simulink model "hw1_suspension"  (R2019b)
settings: Solver=ode1  StartTime=0.0  StopTime=7  FixedStep=0.01  RelTol=1e-3
settings Model: Creator=mahdie  LastModifiedBy=mahdie

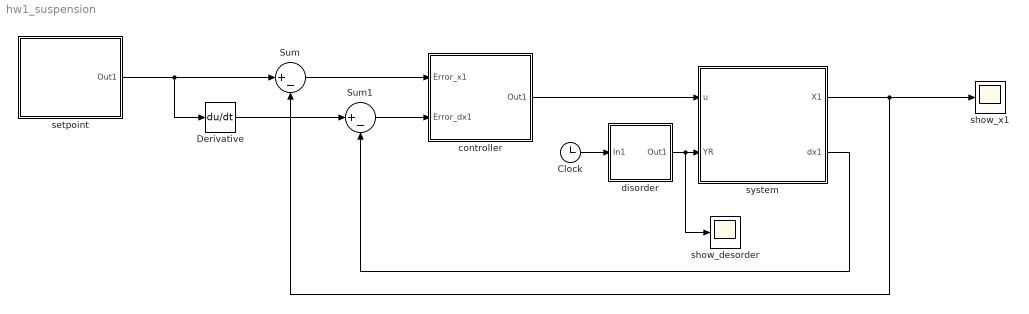
== system hw1_suspension ==
  Clock : Clock
  Derivative : Derivative
  Sum : Sum  Inputs=|+-
  Sum1 : Sum  Inputs=|+-
  controller : Subsystem
  disorder : Subsystem
  "setpoint " : Subsystem
  show_desorder : Scope
  show_x1 : Scope
  "system " : Subsystem
  wires:
  controller/1(Out1) -> "system "/1("u ")
  "system "/1("X1 ") -> show_x1/1, Sum/2
  Sum/1 -> controller/1(Error_x1)
  "setpoint "/1(Out1) -> Derivative/1, Sum/1
  "system "/2("dx1 ") -> Sum1/2
  Sum1/1 -> controller/2(Error_dx1)
  Derivative/1 -> Sum1/1
  Clock/1 -> disorder/1(In1)
  disorder/1(Out1) -> show_desorder/1, "system "/2("YR ")

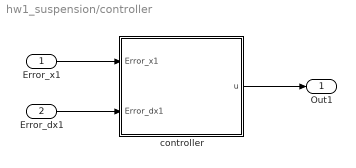
== system hw1_suspension/controller ==
  Error_x1 : Inport
  Error_dx1 : Inport  Port=2
  controller : MATLAB Function  TreatAsAtomicUnit=on
  Out1 : Outport
  wires:
  controller/1(u) -> Out1/1
  Error_x1/1 -> controller/1(Error_x1)
  Error_dx1/1 -> controller/2(Error_dx1)

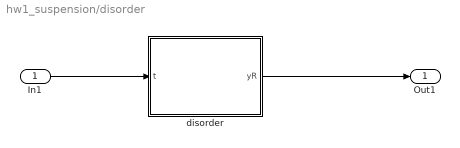
== system hw1_suspension/disorder ==
  In1 : Inport
  disorder : MATLAB Function  TreatAsAtomicUnit=on
  Out1 : Outport
  wires:
  disorder/1(yR) -> Out1/1
  In1/1 -> disorder/1(t)

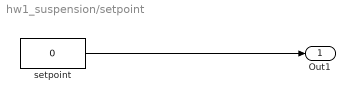
== system hw1_suspension/setpoint  ==
  "setpoint " : Constant  Value=0
  Out1 : Outport
  wires:
  "setpoint "/1 -> Out1/1

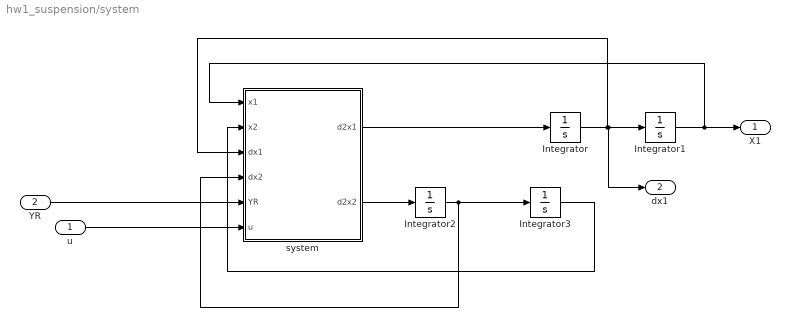
== system hw1_suspension/system  ==
  "u " : Inport
  "YR " : Inport  Port=2
  Integrator : Integrator
  Integrator1 : Integrator  InitialCondition=0.20
  Integrator2 : Integrator
  Integrator3 : Integrator
  "system " : MATLAB Function  TreatAsAtomicUnit=on
  "X1 " : Outport
  "dx1 " : Outport  Port=2
  wires:
  Integrator/1 -> "system "/3(dx1), "dx1 "/1, Integrator1/1
  "system "/2(d2x2) -> Integrator2/1
  Integrator2/1 -> "system "/4(dx2), Integrator3/1
  "system "/1(d2x1) -> Integrator/1
  Integrator1/1 -> "system "/1(x1), "X1 "/1
  Integrator3/1 -> "system "/2(x2)
  "YR "/1 -> "system "/5(YR)
  "u "/1 -> "system "/6(u)

== matlab function hw1_suspension/controller/controller ==
  data: Error_x1 input; u output; Error_dx1 input
%%%%%%%%%%%%%%%%%%%%%%%%%%%%%%%%%%%%%%%%%%%%%%%%%%%%%%%%%%%%
% This program was created by the
% matlab R2019b
% 
% 
% 
% Project : suspension
% Date    : 10/24/2020
% Author  : Mahdie Ahmadi & Zahra Karimi
% Company : Isfahan university of technology
% Comments: this function controll the car suspension system
% 
% 
% Program type            : simulation
%%%%%%%%%%%%%%%%%%%%%%%%%%%%%%%%%%%%%%%%%%%%%%%%%%%%%%%%%%

function u = fcn(Error_x1 , Error_dx1)

%%%%%%%%%%%%%%%%%%%%%%%%%  constans  %%%%%%%%%%%%%%%%%%%%%
 Kp = 300; %% proportionality coefficient
 Kd = 300; %% Derivative coefficient

u = Kp*Error_x1 + Kd*Error_dx1; %% control signal

== matlab function hw1_suspension/system /system  ==
  data: x1 input; d2x1 output; x2 input; dx1 input; dx2 input; YR input; d2x2 output; u input
%%%%%%%%%%%%%%%%%%%%%%%%%%%%%%%%%%%%%%%%%%%%%%%%%%%%%%%%%%%%
% This program was created by the
% matlab R2019b
% 
% 
% 
% Project : suspension
% Date    : 10/24/2020
% Author  : Mahdie Ahmadi & Zahra Karimi
% Company : Isfahan university of technology
% Comments: this function discribe the car suspension model
% 
% 
% Program type            : simulation
%%%%%%%%%%%%%%%%%%%%%%%%%%%%%%%%%%%%%%%%%%%%%%%%%%%%%%%%%%

function [d2x1,d2x2 ] = fcn(x1,x2,dx1,dx2,YR , u)
%%%%%%%%%%%%%%%%%%%%%%%% constants  %%%%%%%%%%%%%%%%%%%%%%%
M = 300; %% weight of car (kg)
m = 50; %% weight of tire (kg)
K1 = 3000; %%spring constant (n/m)
K2 = 30000; %%spring constant of tire (n/m)
D = 600; %%Damper conatant (ns/m)

d2x1 = (1/M)*(u-K1*(x1-x2)-D*(dx1-dx2)); %% The second derivative of x1
d2x2 = (1/m)*(-u-K1*(x2-x1)-D*(dx2-dx1)-K2*(x2-YR));%% The second derivative of x2

== matlab function hw1_suspension/disorder/disorder ==
  data: t input; yR output
%%%%%%%%%%%%%%%%%%%%%%%%%%%%%%%%%%%%%%%%%%%%%%%%%%%%%%%%%%%%
% This program was created by the
% matlab R2019b
% 
% 
% 
% Project : suspension
% Date    : 10/24/2020
% Author  : Mahdie Ahmadi & Zahra Karimi
% Company : Isfahan university of technology
% Comments: this function simulatores road fluctuations and ascillations on
% the car body
% 
% 
% Program type            : simulation
%%%%%%%%%%%%%%%%%%%%%%%%%%%%%%%%%%%%%%%%%%%%%%%%%%%%%%%%%%

function yR = fcn(t)

yR = 0.1*(sin(5*t)+sin(9*t)+sin(13*t)+sin(17*t)+sin(21*t)); %% fluctuations of the road

%%yR = 0; %% road without fluctuation
